simulink subsystem "SCIOutAbstractionFocQep"  (R2024b)
settings: Solver=VariableStepAuto  StartTime=0.0  StopTime=10.0  RelTol=1e-3
values from neighbouring files (symbols this model uses):
  dataType = 'single'    [mchp_pmsm_foc_smo_dsPIC33_data.m]
libraries: svdutilitieslib x1
settings Model: Creator=The MathWorks, Inc.  LastModifiedBy=I67977
settings RTWCC: GPUComputeCapability=3.5

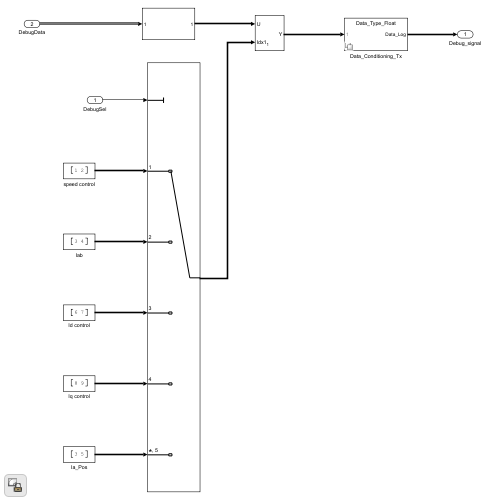
[thumbnail: Simulink's stored preview of the top-level diagram]
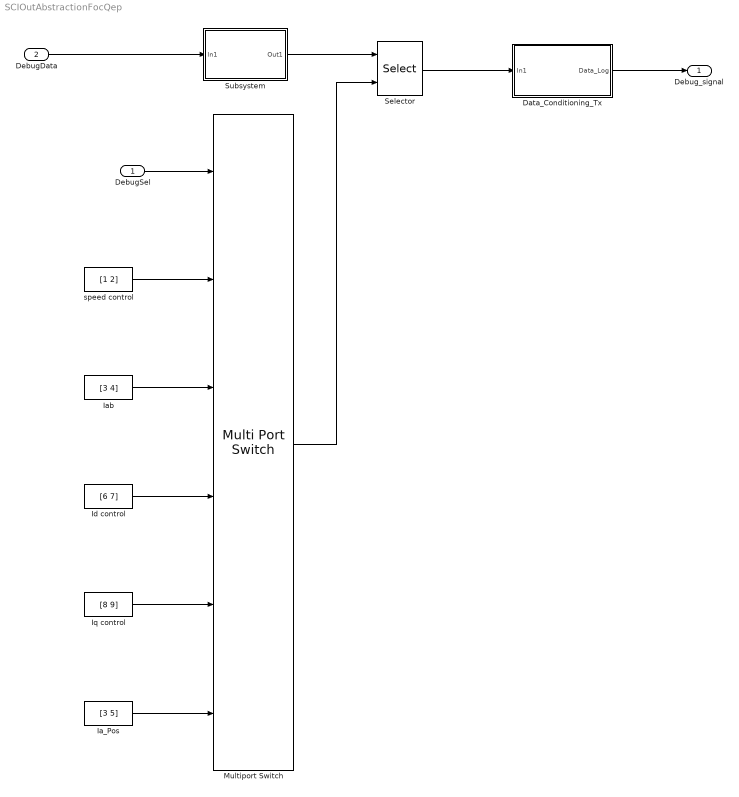
== system SCIOutAbstractionFocQep ==
  DebugSel : Inport
  DebugData : Inport  Port=2
  Data_Conditioning_Tx : Subsystem  Variant=on
  Ia_Pos : Constant  Value=[3 5]  OutDataTypeStr=uint16  SampleTime=-1
  Iab : Constant  Value=[3 4]  OutDataTypeStr=uint16  SampleTime=-1
  Id control : Constant  Value=[6 7]  OutDataTypeStr=uint16  SampleTime=-1
  Iq control : Constant  Value=[8 9]  OutDataTypeStr=uint16  SampleTime=-1
  Multiport Switch : MultiPortSwitch  Inputs=5  DiagnosticForDefault=None  OutDataTypeStr=uint16  RndMeth=Simplest  SaturateOnIntegerOverflow=off  InputSameDT=off
  Selector : Selector  InputPortWidth=11  IndexOptions=Index vector (port)  Indices=[1 3]  OutputSizes=1
  Subsystem : Subsystem
  speed control : Constant  Value=[1 2]  OutDataTypeStr=uint16  SampleTime=-1
  Debug_signal : Outport
  wires:
  speed control/1 -> Multiport Switch/2
  Multiport Switch/1 -> Selector/2
  DebugSel/1 -> Multiport Switch/1
  Data_Conditioning_Tx/1(Data_Log) -> Debug_signal/1
  Iab/1 -> Multiport Switch/3
  DebugData/1 -> Subsystem/1(In1)
  Subsystem/1(Out1) -> Selector/1
  Ia_Pos/1 -> Multiport Switch/6
  Id control/1 -> Multiport Switch/4
  Iq control/1 -> Multiport Switch/5
  Selector/1 -> Data_Conditioning_Tx/1(In1)

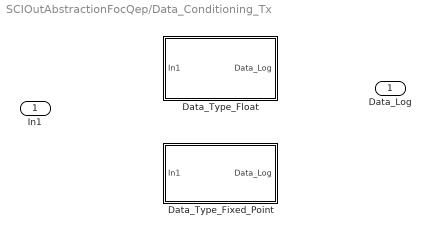
== system SCIOutAbstractionFocQep/Data_Conditioning_Tx ==
  In1 : Inport
  Data_Type_Fixed_Point : Subsystem  VariantControl=~isequal(dataType,'single')
  Data_Type_Float : Subsystem  VariantControl=isequal(dataType, 'single')
  Data_Log : Outport

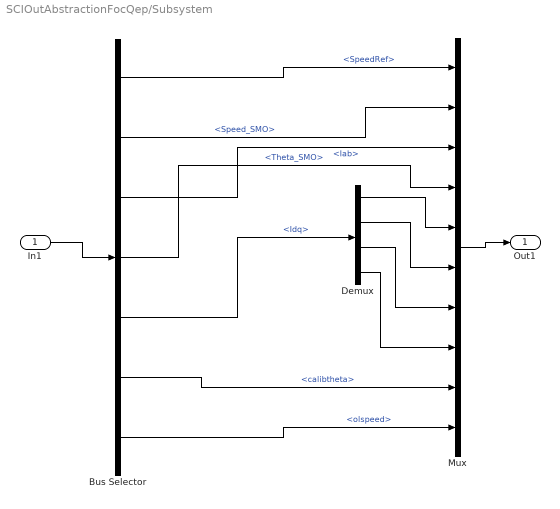
== system SCIOutAbstractionFocQep/Subsystem ==
  In1 : Inport
  Bus Selector : BusSelector  OutputSignals=SpeedRef,Speed_SMO,Iab,Theta_SMO,Idq,calibtheta,olspeed
  Demux : Demux
  Mux : Mux  Inputs=10
  Out1 : Outport
  wires:
  Bus Selector/4 -> Mux/4  "<Theta_SMO>"
  Bus Selector/7 -> Mux/10  "<olspeed>"
  Bus Selector/6 -> Mux/9  "<calibtheta>"
  Bus Selector/2 -> Mux/2  "<Speed_SMO>"
  Demux/4 -> Mux/8
  Demux/3 -> Mux/7
  Demux/2 -> Mux/6
  Demux/1 -> Mux/5
  Bus Selector/5 -> Demux/1  "<Idq>"
  Bus Selector/3 -> Mux/3  "<Iab>"
  Bus Selector/1 -> Mux/1  "<SpeedRef>"
  Mux/1 -> Out1/1
  In1/1 -> Bus Selector/1

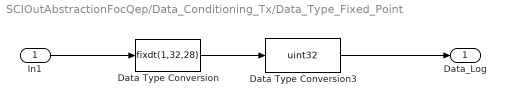
== system SCIOutAbstractionFocQep/Data_Conditioning_Tx/Data_Type_Fixed_Point ==
  In1 : Inport
  Data Type Conversion : DataTypeConversion  OutDataTypeStr=fixdt(1,32,28)  RndMeth=Simplest  SaturateOnIntegerOverflow=off
  Data Type Conversion3 : DataTypeConversion  OutDataTypeStr=uint32  ConvertRealWorld=Stored Integer (SI)  RndMeth=Simplest  SaturateOnIntegerOverflow=off
  Data_Log : Outport
  wires:
  Data Type Conversion/1 -> Data Type Conversion3/1
  Data Type Conversion3/1 -> Data_Log/1
  In1/1 -> Data Type Conversion/1

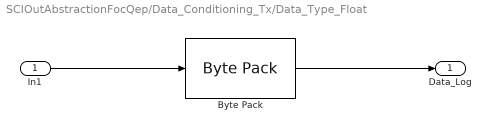
== system SCIOutAbstractionFocQep/Data_Conditioning_Tx/Data_Type_Float ==
  In1 : Inport
  Byte Pack : svdutilitieslib/Byte Pack  maskPackedDataType=uint8  datatypes={'single'}  byteAlign=4  blockPlatform=tic2000
  Data_Log : Outport
  wires:
  In1/1 -> Byte Pack/1
  Byte Pack/1 -> Data_Log/1
